simulink model "two_levelsvpwm"  (R2016a)
settings: Solver=VariableStepAuto  StartTime=0.0  StopTime=0.5  RelTol=1e-3
libraries: powerlib x21, simulink x3
settings Model: Creator=hakan  LastModifiedBy=hakan
settings DataIOCC: LimitDataPoints=on
settings DebuggingCC: AllowSymbolicDim=off
settings ModelReferenceCC: PropagateSignalLabelsOutOfModel=off
settings GRTTargetCC: GeneratePreprocessorConditionals=Use local settings

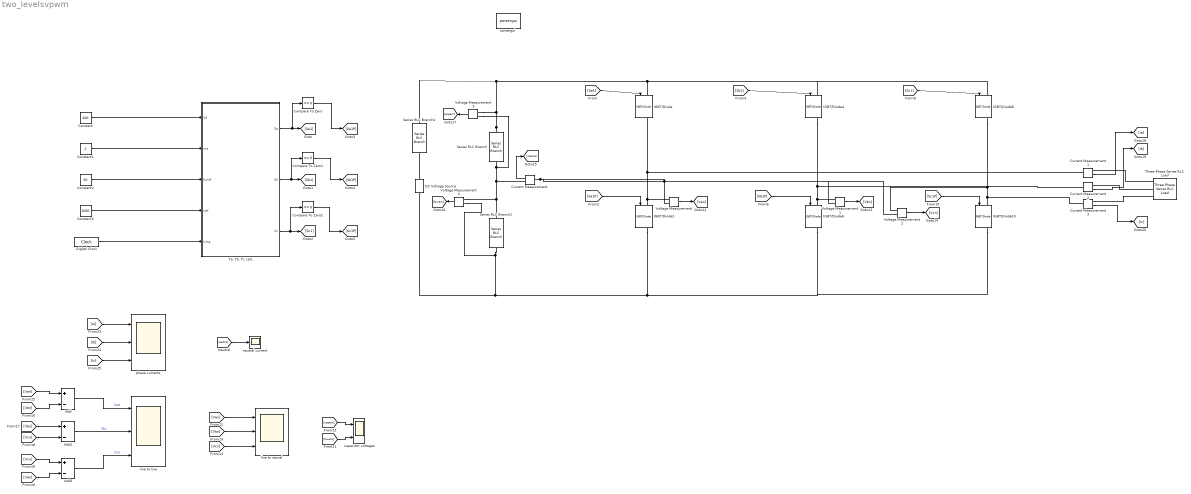
== system two_levelsvpwm ==
  Add : Sum  Inputs=+-
  Add1 : Sum  Inputs=+-
  Add2 : Sum  Inputs=+-
  Compare To Zero : simulink/Logic and Bit Operations/Compare To Zero  relop===  OutDataTypeStr=boolean
  Compare To Zero1 : simulink/Logic and Bit Operations/Compare To Zero  relop===  OutDataTypeStr=boolean
  Compare To Zero2 : simulink/Logic and Bit Operations/Compare To Zero  relop===  OutDataTypeStr=boolean
  Constant : Constant  Value=200
  Constant1 : Constant
  Constant2 : Constant  Value=50
  Constant3 : Constant  Value=1050  VectorParams1D=off
  Current Measurement{,1..3} (4 alike) : powerlib/Measurements/Current Measurement  PhasorSimulation=off  OutputType=Complex  PSBequivalent=0
  DC Voltage Source : powerlib/Electrical Sources/DC Voltage Source  Amplitude=540  Measurements=None
  Digital Clock : DigitalClock  SampleTime=0.0000001
  IGBT/Diode{,2,4,6,8,10} (6 alike) : powerlib/Power Electronics/IGBT//Diode  Ron=1e-3  Rs=1e5  Cs=inf  Measurements=on
  Series RLC Branch : powerlib/Elements/Series RLC Branch  LConnTagsString=__new0  RConnTagsString=__new0  BranchType=C  Resistance=1  Inductance=1e-3  SetiL0=off  InitialCurrent=0  Capacitance=1000e-6  Setx0=off  InitialVoltage=0  Measurements=None
  Series RLC Branch1 : powerlib/Elements/Series RLC Branch  LConnTagsString=__new0  RConnTagsString=__new0  BranchType=C  Resistance=1  Inductance=1e-3  SetiL0=off  InitialCurrent=0  Capacitance=1000e-6  Setx0=off  InitialVoltage=0  Measurements=None
  Series RLC Branch2 : powerlib/Elements/Series RLC Branch  LConnTagsString=__new0  RConnTagsString=__new0  BranchType=R  Resistance=1  Inductance=1e-3  SetiL0=off  InitialCurrent=0  Capacitance=1000e-6  Setx0=off  InitialVoltage=0  Measurements=None
  "Ta, Tb, Tc calc" : MATLAB Function  TreatAsAtomicUnit=on
  Three-Phase Series RLC Load : powerlib/Elements/Three-Phase Series RLC Load  LConnTagsString=A|B|C  Configuration=Y (floating)  NominalVoltage=1000  Vabc=[1e3 1e3 1e3]  Vabcp=[1e3 1e3 1e3]  NominalFrequency=50  UnbalancedPower=off  ActivePower=8000  InductivePower=3870  CapacitivePower=0  Pabc=[10e3 9e3 11e3]  QLabc=[100 90 110]  QCabc=[100 90 110]  Pabcp=[10e3 9e3 11e3]  QLabcp=[100 90 110]  QCabcp=[100 90 110]  Measurements=None  LoadType=constant Z
  Voltage Measurement{,1..4} (5 alike) : powerlib/Measurements/Voltage Measurement  PhasorSimulation=off  OutputType=Complex  PSBequivalent=0
  capacitor voltages : Scope  NumInputPorts=2
  line to line : Scope  NumInputPorts=3
  line to neural : Scope  NumInputPorts=3
  neutral current : Scope
  phase currents : Scope  NumInputPorts=3
  powergui : powerlib/powergui  Priority=1  SimulationMode=Continuous  SolverType=Tustin/Backward Euler (TBE)  SampleTime=50e-6  frequency=60  SPID=off  DisableSnubberDevices=off  DisableRonSwitches=off  DisableVfSwitches=off  SwTol=0  DisplayEquations=off  Interpol=off  ExternalGateDelay=off  methode=off  Ts=10  FunctionMessages=off  echomessages=off  HookPort=off  EnableUseOfTLC=off  x0status=blocks  frequencyindice=0  Pbase=100e6  ErrMax=1e-4  Iterations=50  UnitsV=kV  UnitsW=MW  buscounter=0  RestoreLinks=warning  ResistiveCurrentMeasurement=off  Frange=[0:2:500]  Ylog=off  Xlog=on  ShowGrid=off  save=off  variable=ZData  structure=linetoline  ZoomFFT=off  StartTime=0.0  cycles=2  DisplayStyle=1  fundamental=50  FreqAxis=off  MaxFrequency=5000  frequencyindicesteady=1  RmsSteady=1  display=off
  wires:
  "Ta, Tb, Tc calc"/1(Sa) -> Compare To Zero/1, [Sa1]
  "Ta, Tb, Tc calc"/2(Sb) -> Compare To Zero1/1, [Sb1]
  "Ta, Tb, Tc calc"/3(Sc) -> Compare To Zero2/1, [Sc1]
  Compare To Zero/1 -> [Sa1P]
  Compare To Zero1/1 -> [Sb1P]
  Compare To Zero2/1 -> [Sc1P]
  Constant/1 -> "Ta, Tb, Tc calc"/1(Vd)
  Constant1/1 -> "Ta, Tb, Tc calc"/2(ma)
  Constant2/1 -> "Ta, Tb, Tc calc"/3(fundf)
  Constant3/1 -> "Ta, Tb, Tc calc"/4(swf)
  Digital Clock/1 -> "Ta, Tb, Tc calc"/5(time)
  [Ineutral] -> neutral current/1
  [Ib] -> phase currents/2
  [Ia] -> phase currents/1
  [Ic] -> phase currents/3
  [Van] -> Add/1
  [Vbn] -> Add/2
  Add/1 -> line to line/1  "Vab"
  [Vbn] -> Add1/1
  [Vcn] -> Add1/2
  Add1/1 -> line to line/2  "Vbc"
  [Vcn] -> Add2/1
  [Van] -> Add2/2
  Add2/1 -> line to line/3  "Vca"
  [Van] -> line to neural/1
  [Vbn] -> line to neural/2
  [Vcn] -> line to neural/3
  [lowerc] -> capacitor voltages/2
  [upperc] -> capacitor voltages/1
  [Sa1] -> IGBT/Diode/1
  [Sa1P] -> IGBT/Diode2/1
  [Sb1] -> IGBT/Diode4/1
  [Sb1P] -> IGBT/Diode6/1
  [Sc1] -> IGBT/Diode8/1
  [Sc1P] -> IGBT/Diode10/1
  Voltage Measurement/1 -> [Van]
  Voltage Measurement1/1 -> [Vbn]
  Voltage Measurement2/1 -> [Vcn]
  Voltage Measurement3/1 -> [upperc]
  Voltage Measurement4/1 -> [lowerc]
  Current Measurement/1 -> [Ineutral]
  Current Measurement1/1 -> [Ia]
  Current Measurement2/1 -> [Ib]
  Current Measurement3/1 -> [Ic]
  connections:
  Series RLC Branch/LConn1 -- Voltage Measurement3/LConn1 -- Series RLC Branch2/LConn1 -- IGBT/Diode/LConn1 -- IGBT/Diode4/LConn1 -- IGBT/Diode8/LConn1
  Voltage Measurement4/LConn2 -- Series RLC Branch1/RConn1 -- DC Voltage Source/LConn1 -- IGBT/Diode2/RConn1 -- IGBT/Diode10/RConn1 -- IGBT/Diode6/RConn1
  Current Measurement1/LConn1 -- IGBT/Diode/RConn1 -- IGBT/Diode2/LConn1 -- Voltage Measurement/LConn1
  Current Measurement/LConn1 -- Voltage Measurement/LConn2 -- Voltage Measurement2/LConn2 -- Voltage Measurement1/LConn2
  Current Measurement2/LConn1 -- IGBT/Diode4/RConn1 -- IGBT/Diode6/LConn1 -- Voltage Measurement1/LConn1
  Voltage Measurement2/LConn1 -- IGBT/Diode10/LConn1 -- Current Measurement3/LConn1 -- IGBT/Diode8/RConn1
  Voltage Measurement3/LConn2 -- Series RLC Branch/RConn1 -- Current Measurement/RConn1 -- Series RLC Branch1/LConn1 -- Voltage Measurement4/LConn1
  Three-Phase Series RLC Load/LConn3 -- Current Measurement3/RConn1
  Three-Phase Series RLC Load/LConn1 -- Current Measurement1/RConn1
  Three-Phase Series RLC Load/LConn2 -- Current Measurement2/RConn1
  DC Voltage Source/RConn1 -- Series RLC Branch2/RConn1

== matlab function two_levelsvpwm/Ta, Tb, Tc calc ==
  data: Sa output; Sb output; Vd input; ma input; fundf input; swf input; time input; Sc output
function [Sa, Sb, Sc] = fcn(Vd,ma,fundf, swf, time)
% this program works for magnitude of Vref is greater then Vd/3 meaning ma
% must be greater than 1/sqrt(3). for smaller ma's computation is a bit
% more tricky therefore it is omitted for simplicity for now. 
Vref = ma*Vd/sqrt(3); %magnitude of Vref
theta = 2*pi*fundf*time; %angle of Vref
angle = mod(theta, 2*pi);
Ts = 1/swf;
Ta = 0;
Tb = 0;
Tc = 0;
T0 = 0;
n=0;
output = 0;
%Sector1 = 0; Sector2 = 0; Sector3 = 0; Sector4= 0; Sector5 = 0; Sector6 = 0;
Sa=0; Sb=0; Sc=0;
timee = mod(time,Ts);



%% Sector 1
if (mod(theta, 2*pi)<=pi/3)&&(mod(theta, 2*pi)>0)  % sector 1
    n = 1;
    thetaprime = angle - (n-1)*pi/3;
    
    Ta = Ts*ma*sin(pi/3-thetaprime);
    Tb = Ts*ma*sin(thetaprime);
    T0 = Ts-Ta-Tb;
    
    times = [T0/4 Ta/2 Tb/2 T0/2 Tb/2 Ta/2 T0/4];
    times = cumsum(times);
    va= [0 1 1 1 1 1 0];
    vb= [0 0 1 1 1 0 0];
    vc= [0 0 0 1 0 0 0];
    
    for j = 1:7            
            if(timee<times(j))
                break
            end
    end
        Sa=va(j); 
        Sb=vb(j); 
        Sc=vc(j); 
end
%% Sector 2
if (mod(theta, 2*pi)<=2*pi/3)&&(mod(theta, 2*pi)>pi/3)  % sector 2
    n = 2;
    thetaprime = angle - (n-1)*pi/3;
    
    Ta = Ts*ma*sin(thetaprime);
    Tb = Ts*ma*sin(pi/3-thetaprime);
    T0 = Ts-Ta-Tb;   
    
    times = [T0/4 Ta/2 Tb/2 T0/2 Tb/2 Ta/2 T0/4];
    times = cumsum(times);
    va= [0 0 1 1 1 0 0];
    vb= [0 1 1 1 1 1 0];
    vc= [0 0 0 1 0 0 0];
    
    for j = 1:7            
            if(timee<times(j))
                break
            end
    end
        Sa=va(j); 
        Sb=vb(j); 
        Sc=vc(j); 
end


%% Sector 3
if (mod(theta, 2*pi)<=pi)&&(mod(theta, 2*pi)>2*pi/3)  % sector 3
    n = 3;
    thetaprime = angle - (n-1)*pi/3;
    
    Ta = Ts*ma*sin(pi/3-thetaprime);
    Tb = Ts*ma*sin(thetaprime);
    T0 = Ts-Ta-Tb;  
    
    times = [T0/4 Ta/2 Tb/2 T0/2 Tb/2 Ta/2 T0/4];
    times = cumsum(times);
    va= [0 0 0 1 0 0 0];
    vb= [0 1 1 1 1 1 0];
    vc= [0 0 1 1 1 0 0];
    
    for j = 1:7            
            if(timee<times(j))
                break
            end
    end
        Sa=va(j); 
        Sb=vb(j); 
        Sc=vc(j);     
end


%% Sector 4
if (mod(theta, 2*pi)<=4*pi/3)&&(mod(theta, 2*pi)>pi)  % sector 4
    n = 4;
    thetaprime = angle - (n-1)*pi/3;
    
    Ta = Ts*ma*sin(thetaprime);
    Tb = Ts*ma*sin(pi/3-thetaprime);
    T0 = Ts-Ta-Tb;
    
    times = [T0/4 Ta/2 Tb/2 T0/2 Tb/2 Ta/2 T0/4];
    times = cumsum(times);
    va = [0 0 0 1 0 0 0];
    vb = [0 0 1 1 1 0 0];
    vc = [0 1 1 1 1 1 0];
    
    for j = 1:7            
            if(timee<times(j))
                break
            end
    end
        Sa=va(j); 
        Sb=vb(j); 
        Sc=vc(j); 
    
end


%% Sector 5 
if (mod(theta, 2*pi)<=5*pi/3)&&(mod(theta, 2*pi)>4*pi/3)  % sector 5
    n = 5;
    thetaprime = angle - (n-1)*pi/3;
    
    Ta = Ts*ma*sin(pi/3-thetaprime);
    Tb = Ts*ma*sin(thetaprime);
    T0 = Ts-Ta-Tb;
    
    times = [T0/4 Ta/2 Tb/2 T0/2 Tb/2 Ta/2 T0/4];
    times = cumsum(times);
    va= [0 0 1 1 1 0 0];
    vb= [0 0 0 1 0 0 0];
    vc= [0 1 1 1 1 1 0];
    
    for j = 1:7            
            if(timee<times(j))
                break
            end
    end
        Sa=va(j); 
        Sb=vb(j); 
        Sc=vc(j); 
    
end


%% Sector 6 
if (mod(theta, 2*pi)<=2*pi)&&(mod(theta, 2*pi)>5*pi/3)  % sector 6
    n = 6;
    thetaprime = angle - (n-1)*pi/3;
    
    Ta = Ts*ma*sin(thetaprime);
    Tb = Ts*ma*sin(pi/3-thetaprime);
    T0 = Ts-Ta-Tb;
    
    times = [T0/4 Ta/2 Tb/2 T0/2 Tb/2 Ta/2 T0/4];
    times = cumsum(times);
    va= [0 1 1 1 1 1 0];
    vb= [0 0 0 1 0 0 0];
    vc= [0 0 1 1 1 0 0];
    
    
    for j = 1:7            
            if(timee<times(j))
                break
            end
    end
        Sa=va(j); 
        Sb=vb(j); 
        Sc=vc(j); 
end
